simulink model "led_control_with_detect_change"  (R2025a)
settings: Solver=FixedStepDiscrete  StartTime=0.0  StopTime=20  FixedStep=1  RelTol=1e-3
libraries: simulink x3
settings Model: Creator=mahij  LastModifiedBy=mahij

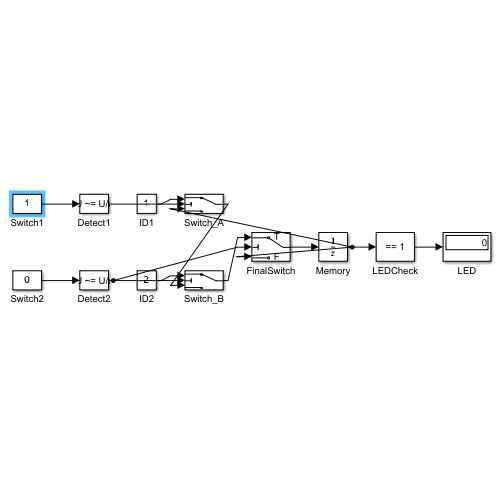
[thumbnail: Simulink's stored preview of the top-level diagram]
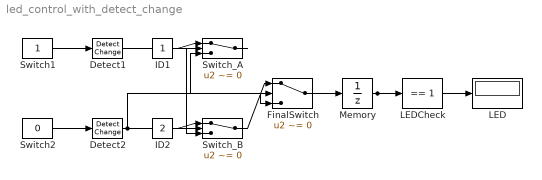
== system led_control_with_detect_change ==
  Detect1 : simulink/Logic and Bit Operations/Detect Change  vinit=0  OutDataTypeStr=boolean
  Detect2 : simulink/Logic and Bit Operations/Detect Change  vinit=0  OutDataTypeStr=boolean
  FinalSwitch : Switch  Criteria=u2 ~= 0  Threshold=0.5  SaturateOnIntegerOverflow=off  InputSameDT=off
  ID1 : Constant
  ID2 : Constant  Value=2
  LED : Display
  LEDCheck : simulink/Logic and Bit Operations/Compare To Constant  relop===  const=1  OutDataTypeStr=boolean
  Memory : UnitDelay  HasFrameUpgradeWarning=on
  Switch1 : Constant
  Switch2 : Constant  Value=0
  Switch_A : Switch  Criteria=u2 ~= 0  Threshold=0.5  SaturateOnIntegerOverflow=off  InputSameDT=off
  Switch_B : Switch  Criteria=u2 ~= 0  Threshold=0.5  SaturateOnIntegerOverflow=off  InputSameDT=off
  wires:
  Switch1/1 -> Detect1/1
  Switch2/1 -> Detect2/1
  ID1/1 -> Switch_A/1
  Detect1/1 -> Switch_A/2
  Memory/1 -> Switch_A/3, FinalSwitch/3, LEDCheck/1
  ID2/1 -> Switch_B/1
  Detect2/1 -> Switch_B/2, FinalSwitch/2
  Switch_A/1 -> Switch_B/3
  Switch_B/1 -> FinalSwitch/1
  FinalSwitch/1 -> Memory/1
  LEDCheck/1 -> LED/1
